simulink model "KITTDynamics"  (R2014b)
settings: Solver=ode45  StartTime=0.0  StopTime=8.0  MaxStep=0.01  RelTol=1e-3
values from neighbouring files (symbols this model uses):
  b = 0.0015    [KITTParameters.m]
  c = 0.002    [KITTParameters.m]
  m = 13    [KITTParameters.m]
undefined symbols (not defined in the file or in its folder): Fa, Fb, V_ini
settings Model: Creator=Martijn  LastModifiedBy=Martijn
settings DataIOCC: LimitDataPoints=off

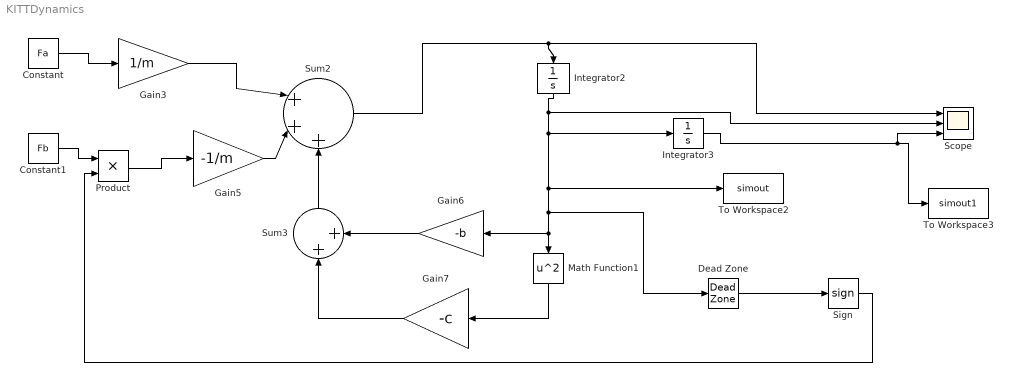
== system KITTDynamics ==
  Constant : Constant  Value=Fa
  Constant1 : Constant  Value=Fb
  Dead Zone : DeadZone  LowerValue=-0.001  UpperValue=0.001  SaturateOnIntegerOverflow=on
  Gain3 : Gain  Gain=1/m
  Gain5 : Gain  Gain=-1/m
  Gain6 : Gain  Gain=-b
  Gain7 : Gain  Gain=-c
  Integrator2 : Integrator  InitialCondition=V_ini
  Integrator3 : Integrator
  Math Function1 : Math  Operator=square  SaturateOnIntegerOverflow=on
  Product : Product
  Scope : Scope  NumInputPorts=3
      settings: YMin=-5~-5~-5  YMax=5~5~5
  Sign : Signum
  Sum2 : Sum  Inputs=|+++
  Sum3 : Sum  Inputs=|++
  "To Workspace2 " : ToWorkspace  VariableName=simout  SaveFormat=Structure With Time  SampleTime=-1
  To Workspace3 : ToWorkspace  VariableName=simout1  SaveFormat=Structure With Time  SampleTime=-1
  wires:
  Gain5/1 -> Sum2/2
  Gain3/1 -> Sum2/1
  Gain6/1 -> Sum3/2
  Sum3/1 -> Sum2/3
  Integrator2/1 -> Scope/2, Integrator3/1, "To Workspace2 "/1, Dead Zone/1, Math Function1/1, Gain6/1
  Math Function1/1 -> Gain7/1
  Sign/1 -> Product/2
  Integrator3/1 -> Scope/3, To Workspace3/1
  Gain7/1 -> Sum3/1
  Sum2/1 -> Scope/1, Integrator2/1
  Product/1 -> Gain5/1
  Dead Zone/1 -> Sign/1
  Constant/1 -> Gain3/1
  Constant1/1 -> Product/1
